simulink model "BlueRov2BacksteppingSMC"  (R2025a)
settings: Solver=ode4  StartTime=0.0  StopTime=30  FixedStep=0.001  RelTol=1e-3
settings Model: Creator=oisin  LastModifiedBy=oisin
settings DataIOCC: ReturnWorkspaceOutputsName=BSSM

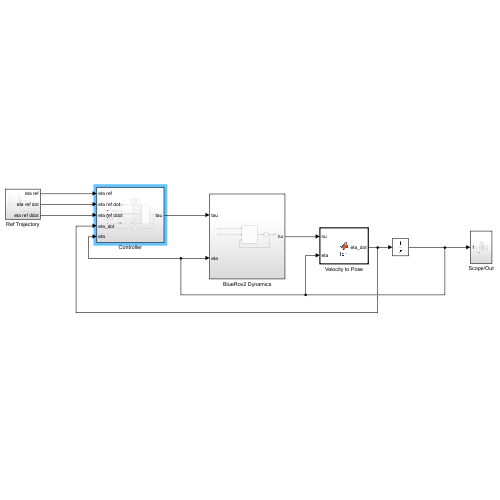
[thumbnail: Simulink's stored preview of the top-level diagram]
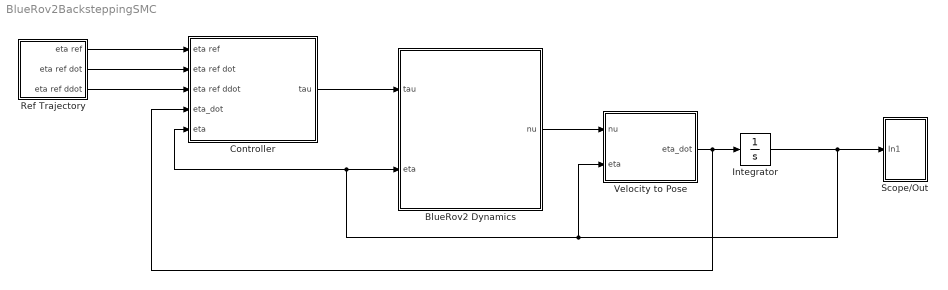
== system BlueRov2BacksteppingSMC ==
  BlueRov2 Dynamics : Subsystem
  Controller : Subsystem
  Integrator : Integrator  InitialCondition=[10;0;0;0;0;0]
  Ref Trajectory : Subsystem
  Scope/Out : Subsystem
  Velocity to Pose : MATLAB Function  TreatAsAtomicUnit=on
  wires:
  Controller/1(tau) -> BlueRov2 Dynamics/1(tau)
  Integrator/1 -> Controller/5(eta), BlueRov2 Dynamics/2(eta), Velocity to Pose/2(eta), Scope/Out/1(In1)
  BlueRov2 Dynamics/1(nu) -> Velocity to Pose/1(nu)
  Velocity to Pose/1(eta_dot) -> Integrator/1, Controller/4(eta_dot)
  Ref Trajectory/1(eta ref) -> Controller/1(eta ref)
  Ref Trajectory/2(eta ref dot) -> Controller/2(eta ref dot)
  Ref Trajectory/3(eta ref ddot) -> Controller/3(eta ref ddot)

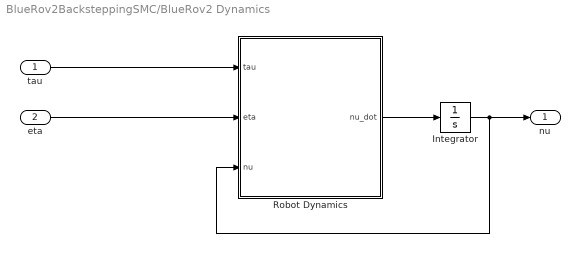
== system BlueRov2BacksteppingSMC/BlueRov2 Dynamics ==
  tau : Inport
  eta : Inport  Port=2
  Integrator : Integrator  InitialCondition=[0;0;0;0;0;0]
  Robot Dynamics : MATLAB Function  TreatAsAtomicUnit=on
  nu : Outport
  wires:
  Robot Dynamics/1(nu_dot) -> Integrator/1
  tau/1 -> Robot Dynamics/1(tau)
  eta/1 -> Robot Dynamics/2(eta)
  Integrator/1 -> nu/1, Robot Dynamics/3(nu)

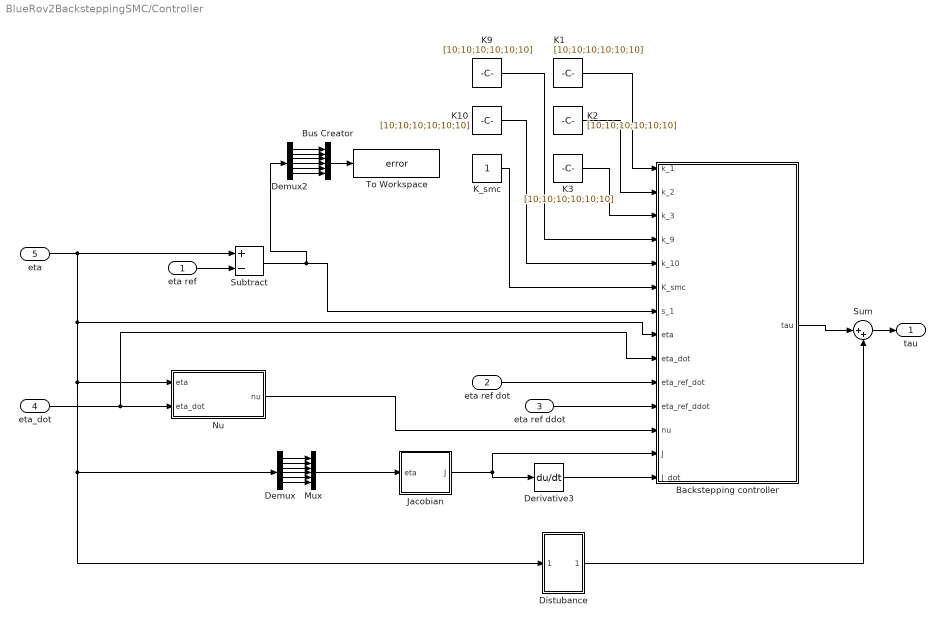
== system BlueRov2BacksteppingSMC/Controller ==
  eta ref : Inport
  eta ref dot : Inport  Port=2
  eta ref ddot : Inport  Port=3
  eta_dot : Inport  Port=4
  eta : Inport  Port=5
  Backstepping controller : MATLAB Function  TreatAsAtomicUnit=on
  Bus Creator : BusCreator  Inputs=6
  Demux : Demux  Outputs=6
  Demux2 : Demux  Outputs=6
  Derivative3 : Derivative
  Distubance : Subsystem
  Jacobian : MATLAB Function  TreatAsAtomicUnit=on
  K{1..3,9..10} (5 alike) : Constant  Value=[10;10;10;10;10;10]
  K_smc : Constant
  Mux : Mux  Inputs=6
  Nu : MATLAB Function  TreatAsAtomicUnit=on
  Subtract : Sum  Inputs=+-
  Sum : Sum  Inputs=|++
  To Workspace : ToWorkspace  VariableName=error  SampleTime=-1
  tau : Outport
  wires:
  eta/1 -> Subtract/1, Distubance/1(eta), Demux/1, Nu/1(eta), Backstepping controller/8(eta)
  eta_dot/1 -> Backstepping controller/9(eta_dot), Nu/2(eta_dot)
  Nu/1(nu) -> Backstepping controller/12(nu)
  Jacobian/1(J) -> Backstepping controller/13(J), Derivative3/1
  Demux/5 -> Mux/5
  Demux/3 -> Mux/3
  Demux/2 -> Mux/2
  Demux/6 -> Mux/6
  Demux/4 -> Mux/4
  Mux/1 -> Jacobian/1(eta)
  Demux/1 -> Mux/1
  Subtract/1 -> Demux2/1, Backstepping controller/7(s_1)
  eta ref dot/1 -> Backstepping controller/10(eta_ref_dot)
  eta ref ddot/1 -> Backstepping controller/11(eta_ref_ddot)
  Derivative3/1 -> Backstepping controller/14(J_dot)
  Backstepping controller/1(tau) -> Sum/1
  Sum/1 -> tau/1
  Distubance/1(Out1) -> Sum/2
  eta ref/1 -> Subtract/2
  K1/1 -> Backstepping controller/1(k_1)
  K2/1 -> Backstepping controller/2(k_2)
  K3/1 -> Backstepping controller/3(k_3)
  K_smc/1 -> Backstepping controller/6(K_smc)
  K10/1 -> Backstepping controller/5(k_10)
  K9/1 -> Backstepping controller/4(k_9)
  Demux2/3 -> Bus Creator/3
  Demux2/2 -> Bus Creator/2
  Demux2/1 -> Bus Creator/1
  Demux2/4 -> Bus Creator/4
  Bus Creator/1 -> To Workspace/1
  Demux2/5 -> Bus Creator/5
  Demux2/6 -> Bus Creator/6

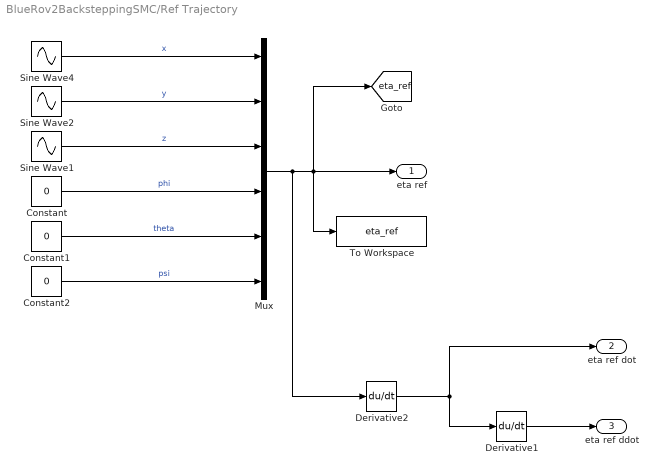
== system BlueRov2BacksteppingSMC/Ref Trajectory ==
  Constant : Constant  Value=0
  Constant1 : Constant  Value=0
  Constant2 : Constant  Value=0
  Derivative1 : Derivative
  Derivative2 : Derivative
  Mux : Mux  Inputs=6
  Sine Wave1 : Sin  Amplitude=5  Bias=-10  Frequency=pi/6  Phase=pi/2  SampleTime=0
  Sine Wave2 : Sin  Amplitude=10  Frequency=(2*pi)/30  SampleTime=0
  Sine Wave4 : Sin  Amplitude=10  Frequency=(2*pi)/30  Phase=pi/2  SampleTime=0
  To Workspace : ToWorkspace  VariableName=eta_ref  SaveFormat=Timeseries  SampleTime=-1
  eta ref : Outport
  eta ref dot : Outport  Port=2
  eta ref ddot : Outport  Port=3
  tag scope: eta_ref=global
  wires:
  Sine Wave4/1 -> Mux/1  "x"
  Constant1/1 -> Mux/5  "theta"
  Constant2/1 -> Mux/6  "psi"
  Constant/1 -> Mux/4  "phi"
  Mux/1 -> To Workspace/1, [eta_ref], eta ref/1, Derivative2/1
  Sine Wave1/1 -> Mux/3  "z"
  Sine Wave2/1 -> Mux/2  "y"
  Derivative1/1 -> eta ref ddot/1
  Derivative2/1 -> eta ref dot/1, Derivative1/1

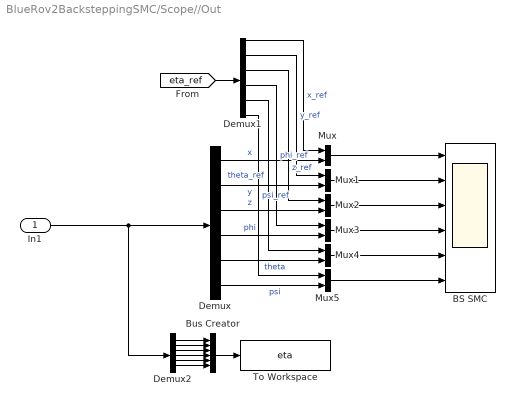
== system BlueRov2BacksteppingSMC/Scope//Out ==
  In1 : Inport
  BS SMC : Scope  NumInputPorts=6
      settings: ActiveDisplayYMinimum=-12.500015260678529  ActiveDisplayYMaximum=12.500137346106756
  Bus Creator : BusCreator  Inputs=6
  Demux : Demux  Outputs=6
  Demux1 : Demux  Outputs=6
  Demux2 : Demux  Outputs=6
  Mux{,1..5} (6 alike) : Mux  Inputs=2
  To Workspace : ToWorkspace  VariableName=eta  SampleTime=-1
  wires:
  Demux/4 -> Mux3/2  "phi"
  Demux1/2 -> Mux1/1  "y_ref"
  [eta_ref] -> Demux1/1
  Mux5/1 -> BS SMC/6
  Demux1/5 -> Mux4/1  "theta_ref"
  Demux/1 -> Mux/2  "x"
  Demux/5 -> Mux4/2  "theta"
  Mux/1 -> BS SMC/1
  Demux/3 -> Mux2/2  "z"
  Mux1/1 -> BS SMC/2
  Mux2/1 -> BS SMC/3
  Demux/2 -> Mux1/2  "y"
  Demux1/6 -> Mux5/1  "psi_ref"
  Mux3/1 -> BS SMC/4
  Demux1/3 -> Mux2/1  "z_ref"
  Mux4/1 -> BS SMC/5
  Demux1/4 -> Mux3/1  "phi_ref"
  Demux/6 -> Mux5/2  "psi"
  Demux1/1 -> Mux/1  "x_ref"
  In1/1 -> Demux2/1, Demux/1
  Demux2/4 -> Bus Creator/4
  Demux2/3 -> Bus Creator/3
  Demux2/1 -> Bus Creator/1
  Demux2/6 -> Bus Creator/6
  Demux2/2 -> Bus Creator/2
  Demux2/5 -> Bus Creator/5
  Bus Creator/1 -> To Workspace/1

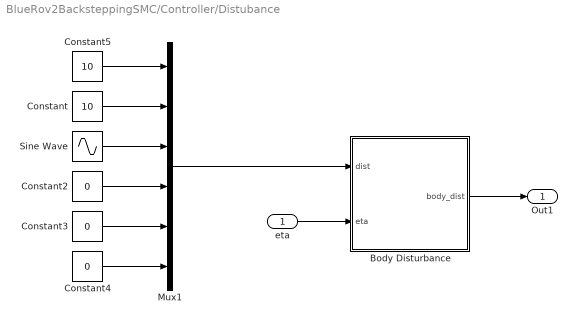
== system BlueRov2BacksteppingSMC/Controller/Distubance ==
  eta : Inport
  Body Disturbance : MATLAB Function  TreatAsAtomicUnit=on
  Constant : Constant  Value=10
  Constant2 : Constant  Value=0
  Constant3 : Constant  Value=0
  Constant4 : Constant  Value=0
  Constant5 : Constant  Value=10
  Mux1 : Mux  Inputs=6
  Sine Wave : Sin  Amplitude=10  SampleTime=0
  Out1 : Outport
  wires:
  Constant2/1 -> Mux1/4
  Constant3/1 -> Mux1/5
  Constant4/1 -> Mux1/6
  Body Disturbance/1(body_dist) -> Out1/1
  Mux1/1 -> Body Disturbance/1(dist)
  eta/1 -> Body Disturbance/2(eta)
  Constant5/1 -> Mux1/1
  Constant/1 -> Mux1/2
  Sine Wave/1 -> Mux1/3

== matlab function BlueRov2BacksteppingSMC/Velocity to Pose ==
  data: nu input; eta_dot output; eta input
function eta_dot = fcn(nu, eta)

eta_dot=zeros(6,1);

phi   = eta(4);
theta = eta(5);
psi   = eta(6);

J=[(cos(psi)*(cos(theta))),((-sin(psi))*(cos(phi)))+((cos(psi))*(sin(theta))*(sin(phi))),((sin(psi))*(sin(phi)))+((cos(psi))*(cos(phi))*(sin(theta))),0,0,0;
    (sin(psi))*(cos(theta)),((cos(psi))*(cos(phi)))+((sin(phi))*(sin(theta))*(sin(psi))),((-cos(psi))*(sin(phi)))+((sin(theta))*(sin(psi))*(cos(phi))),0,0,0;
    -sin(theta),(cos(theta))*(sin(phi)),(cos(theta))*(cos(phi)),0,0,0;
    0,0,0,1,(sin(phi))*(tan(theta)),(cos(phi))*(tan(theta));
    0,0,0,0,cos(phi),-sin(phi);
    0,0,0,0,(sin(phi))/(cos(theta)),(cos(phi))/(cos(theta))];

eta_dot = J * nu;

== matlab function BlueRov2BacksteppingSMC/BlueRov2 Dynamics/Robot Dynamics ==
  data: tau input; nu_dot output; eta input; nu input
function nu_dot = fcn(tau, eta, nu)

nu_dot=zeros(6,1);

t1=tau(1,1);
t2=tau(2,1);
t3=tau(3,1);
t4=tau(4,1);
t5=tau(5,1);
t6=tau(6,1);

tautot=[t1;t2;t3;t4;t5;t6];

m  = 11.5;
W  = 112.8;
B  = 114.8;

Ix = 0.16;
Iy = 0.16;
Iz = 0.16;
zg = 0.0;

X_udot  = -5.5;
Y_vdot  = -12.7;
Z_wdot  = -14.57;
K_pdot  = -0.12;
M_qdot  = -0.12;
N_rdot  = -0.12; 

X_u = -4.03;
Y_v = -6.22;
Z_w = -5.18;
K_p = -0.07;
M_q = -0.07;
N_r = -0.07;

X_uu        = -18.18;
Y_vv        = -21.66;
Z_ww        = -36.99;
K_pp        = -1.55;
M_qq        = -1.55; 
N_rr        = -1.55;  

x=eta(1,1);
y=eta(2,1);
z=eta(3,1);
phi=eta(4,1);
theta=eta(5,1);
psi=eta(6,1);

u=nu(1,1);
v=nu(2,1);
w=nu(3,1);
p=nu(4,1);
q=nu(5,1);
r=nu(6,1);

% mass matrices
M_A = -diag([X_udot,Y_vdot,Z_wdot,K_pdot,M_qdot,N_rdot]);

M_RB = [ m   0    0    0      m*zg  0;
          0   m    0   -m*zg   0     0;
          0   0    m    0      0     0;
          0  -m*zg 0   Ix      0     0;
          m*zg 0   0    0      Iy    0;
          0    0   0    0      0     Iz ];


M_total = M_A + M_RB;

% Coriolis matrices
C_A = [ 0     0     0      0          Z_wdot*w     0;
         0     0     0     -Z_wdot*w  0            -X_udot*u;
         0     0     0      Y_vdot*v   -N_rdot*r    0;
         0     Z_wdot*w  -Y_vdot*v    0            -K_pdot*p   0;
        -Z_wdot*w   0     X_udot*u    K_pdot*p      0          0;
        -Y_vdot*v  X_udot*u   0       0             0          0 ];

C_RB = [ 0     0     0     0     m*w   -m*v;
          0     0     0    -m*w   0      m*u;
          0     0     0     m*v  -m*u    0;
          0    -m*w   m*v   0    Iz*r   -Iy*q;
          m*w   0    -m*u  -Iz*r 0       Ix*p;
         -m*v   m*u   0     Iy*q -Ix*p   0 ];

C_total = C_A + C_RB;

% Restoring forces
g_eta = [ (W - B) * sin(theta);
         -(W - B) * cos(theta) * sin(phi);
         -(W - B) * cos(theta) * cos(phi);
          zg * W * cos(theta) * sin(phi);
          zg * W * sin(theta);
          0 ];

% damping
D_lin = -diag([X_u, Y_v, Z_w, K_p, M_q, N_r]);

D_quad = -diag([X_uu*abs(u), Y_vv*abs(v), Z_ww*abs(w), K_pp*abs(p), M_qq*abs(q), N_rr*abs(r)]);

D_total = D_lin + D_quad;


% calculate nu_dot
nu_dot = M_total \ (tautot-((C_total*nu)+(D_total*nu)+g_eta));

== matlab function BlueRov2BacksteppingSMC/Controller/Backstepping controller ==
  data: k_1 input; k_2 input; k_3 input; k_9 input; k_10 input; K_smc input; s_1 input; eta input; eta_dot input; eta_ref_dot input; eta_ref_ddot input; tau output; nu input; J input; J_dot input
function tau = fcn(k_1, k_2, k_3, k_9, k_10, K_smc, s_1, eta, eta_dot, eta_ref_dot, eta_ref_ddot, nu, J, J_dot)

tau = zeros(6,1);

% constants
alpha = 0.5;
beta = 2;

m  = 11.5;
W  = 112.8;
B  = 114.8;

Ix = 0.16;
Iy = 0.16;
Iz = 0.16;
zg = 0.0;

X_udot  = -5.5;
Y_vdot  = -12.7;
Z_wdot  = -14.57;
K_pdot  = -0.12;
M_qdot  = -0.12;
N_rdot  = -0.12; 

X_u = -4.03;
Y_v = -6.22;
Z_w = -5.18;
K_p = -0.07;
M_q = -0.07;
N_r = -0.07;

X_uu        = -18.18;
Y_vv        = -21.66;
Z_ww        = -36.99;
K_pp        = -1.55;
M_qq        = -1.55; 
N_rr        = -1.55;  

x=eta(1,1);
y=eta(2,1);
z=eta(3,1);
phi=eta(4,1);
theta=eta(5,1);
psi=eta(6,1);

u=nu(1,1);
v=nu(2,1);
w=nu(3,1);
p=nu(4,1);
q=nu(5,1);
r=nu(6,1);

% mass matrices
M_A = -diag([X_udot,Y_vdot,Z_wdot,K_pdot,M_qdot,N_rdot]);

M_RB = [ m   0    0    0      m*zg  0;
          0   m    0   -m*zg   0     0;
          0   0    m    0      0     0;
          0  -m*zg 0   Ix      0     0;
          m*zg 0   0    0      Iy    0;
          0    0   0    0      0     Iz ];


M_hat = M_A + M_RB;

% coriolis matrices
C_A = [ 0     0     0      0          Z_wdot*w     0;
         0     0     0     -Z_wdot*w  0            -X_udot*u;
         0     0     0      Y_vdot*v   -N_rdot*r    0;
         0     Z_wdot*w  -Y_vdot*v    0            -K_pdot*p   0;
        -Z_wdot*w   0     X_udot*u    K_pdot*p      0          0;
        -Y_vdot*v  X_udot*u   0       0             0          0 ];

C_RB = [ 0     0     0     0     m*w   -m*v;
          0     0     0    -m*w   0      m*u;
          0     0     0     m*v  -m*u    0;
          0    -m*w   m*v   0    Iz*r   -Iy*q;
          m*w   0    -m*u  -Iz*r 0       Ix*p;
         -m*v   m*u   0     Iy*q -Ix*p   0 ];

C_hat = C_A + C_RB;

% restoring forces
g_etahat = [ (W - B) * sin(theta);
         -(W - B) * cos(theta) * sin(phi);
         -(W - B) * cos(theta) * cos(phi);
          zg * W * cos(theta) * sin(phi);
          zg * W * sin(theta);
          0 ];

% damping
D_lin = -diag([X_u, Y_v, Z_w, K_p, M_q, N_r]);

D_quad = -diag([X_uu*abs(u), Y_vv*abs(v), Z_ww*abs(w), K_pp*abs(p), M_qq*abs(q), N_rr*abs(r)]);

D_hat = D_lin + D_quad;

%% Backstepping Control

s_1dot = eta_dot - eta_ref_dot;

s_1_alpha = sign(s_1) .* (abs(s_1) .^ alpha);
s_1_beta = sign(s_1) .* (abs(s_1) .^ beta);

alpha_s = J \ (eta_ref_dot - k_1 .* s_1 - k_2 .* s_1_alpha - k_3 .* s_1_beta );

alphadot_s = J\(eta_ref_ddot - ((k_1 .* s_1dot)+(k_2 .* s_1_alpha)+(k_3 .* s_1_beta)) - (J_dot * alpha_s));

s_2 = nu - alpha_s;

%% Slide Mode Control

s_2_alpha = sign(s_2) .* (abs(s_2) .^ alpha);
s_2_beta = sign(s_2) .* (abs(s_2) .^ beta);

% sliding surface
S_S = s_2 + k_9 .* s_2_alpha + k_10 .* s_2_beta;

%k_s = 1.5;

%S_S = sign(k_s * s_1); 

% Define tau limits
max_tau = [88; 88; 137; 23.3; 23.3; 21.6];
tau_unsat = (M_hat*alphadot_s) + (C_hat*nu) + (D_hat*nu) + g_etahat - K_smc * S_S;
% Saturation
tau = max(min(tau_unsat, max_tau), -max_tau);

%tau = (M_hat*alphadot_s) + (C_hat*nu) + (D_hat*nu) + g_etahat - K_smc * S_S;

== matlab function BlueRov2BacksteppingSMC/Controller/Distubance/Body Disturbance ==
  data: dist input; body_dist output; eta input
function body_dist  = fcn(dist,eta)

phi=eta(4,1);
theta=eta(5,1);
psi=eta(6,1);

J=[(cos(psi)*(cos(theta))),((-sin(psi))*(cos(phi)))+((cos(psi))*(sin(theta))*(sin(phi))),((sin(psi))*(sin(phi)))+((cos(psi))*(cos(phi))*(sin(theta))),0,0,0;
    (sin(psi))*(cos(theta)),((cos(psi))*(cos(phi)))+((sin(phi))*(sin(theta))*(sin(psi))),((-cos(psi))*(sin(phi)))+((sin(theta))*(sin(psi))*(cos(phi))),0,0,0;
    -sin(theta),(cos(theta))*(sin(phi)),(cos(theta))*(cos(phi)),0,0,0;
    0,0,0,1,(sin(phi))*(tan(theta)),(cos(phi))*(tan(theta));
    0,0,0,0,cos(phi),-sin(phi);
    0,0,0,0,(sin(phi))/(cos(theta)),(cos(phi))/(cos(theta))];


body_dist= J \ dist;

== matlab function BlueRov2BacksteppingSMC/Controller/Nu ==
  data: eta input; nu output; eta_dot input
function nu = fcn(eta, eta_dot)

nu=zeros(6,1);

phi=eta(4,1);
theta=eta(5,1);
psi=eta(6,1);

J=[(cos(psi)*(cos(theta))),((-sin(psi))*(cos(phi)))+((cos(psi))*(sin(theta))*(sin(phi))),((sin(psi))*(sin(phi)))+((cos(psi))*(cos(phi))*(sin(theta))),0,0,0;
    (sin(psi))*(cos(theta)),((cos(psi))*(cos(phi)))+((sin(phi))*(sin(theta))*(sin(psi))),((-cos(psi))*(sin(phi)))+((sin(theta))*(sin(psi))*(cos(phi))),0,0,0;
    -sin(theta),(cos(theta))*(sin(phi)),(cos(theta))*(cos(phi)),0,0,0;
    0,0,0,1,(sin(phi))*(tan(theta)),(cos(phi))*(tan(theta));
    0,0,0,0,cos(phi),-sin(phi);
    0,0,0,0,(sin(phi))/(cos(theta)),(cos(phi))/(cos(theta))];

nu = J \ eta_dot;

== matlab function BlueRov2BacksteppingSMC/Controller/Jacobian ==
  data: eta input; J output
function J = fcn(eta)

phi   = eta(4);
theta = eta(5);
psi   = eta(6);

J=[(cos(psi)*(cos(theta))),((-sin(psi))*(cos(phi)))+((cos(psi))*(sin(theta))*(sin(phi))),((sin(psi))*(sin(phi)))+((cos(psi))*(cos(phi))*(sin(theta))),0,0,0;
    (sin(psi))*(cos(theta)),((cos(psi))*(cos(phi)))+((sin(phi))*(sin(theta))*(sin(psi))),((-cos(psi))*(sin(phi)))+((sin(theta))*(sin(psi))*(cos(phi))),0,0,0;
    -sin(theta),(cos(theta))*(sin(phi)),(cos(theta))*(cos(phi)),0,0,0;
    0,0,0,1,(sin(phi))*(tan(theta)),(cos(phi))*(tan(theta));
    0,0,0,0,cos(phi),-sin(phi);
    0,0,0,0,(sin(phi))/(cos(theta)),(cos(phi))/(cos(theta))];

end
